simulink model "QcarModel_RoadExcitation_R2023a"  (R2023b)
settings: Solver=FixedStepAuto  StartTime=0.0  StopTime=5  FixedStep=0.01  RelTol=1e-3
values from neighbouring files (symbols this model uses):
  c = 20000    [QCarModel_Frequency_V2.m]    (also in QCarModel_Parameters.m)
  d = 1500    [QCarModel_Frequency_V2.m]    (also in QCarModel_Parameters.m)
  g = 981/100    (= 9.81)    [QCarModel_Frequency_V2.m]    (also in QCarModel_Parameters.m)
  m = mass(h)    [QCarModel_Frequency_V2.m]    (also in QCarModel_Parameters.m = 400)
settings Model: Creator=erona  LastModifiedBy=BeanieBabyJ
settings RTWCC: GPUComputeCapability=5.0

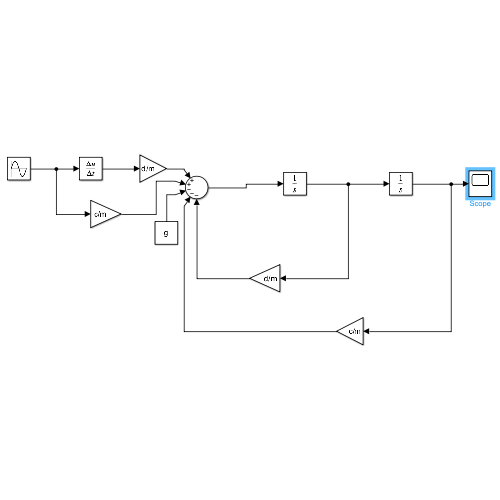
[thumbnail: Simulink's stored preview of the top-level diagram]
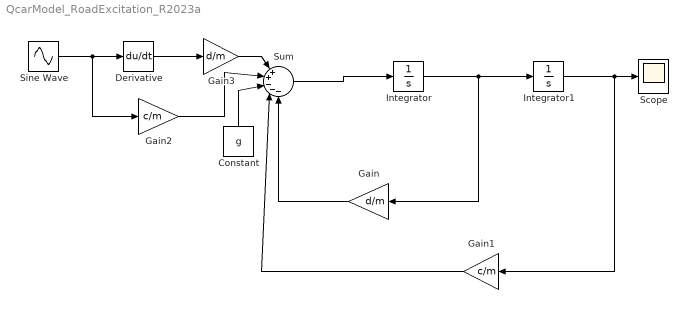
== system QcarModel_RoadExcitation_R2023a ==
  Constant : Constant  Value=g
  Derivative : Derivative
  Gain : Gain  Gain=d/m
  Gain1 : Gain  Gain=c/m
  Gain2 : Gain  Gain=c/m
  Gain3 : Gain  Gain=d/m
  Integrator : Integrator
  Integrator1 : Integrator
  Scope : Scope
  Sine Wave : Sin  Amplitude=0.02  Frequency=2*pi*100  Phase=pi/2  SampleTime=0
  Sum : Sum  Inputs=|++---
  wires:
  Integrator/1 -> Gain/1, Integrator1/1
  Sum/1 -> Integrator/1
  Integrator1/1 -> Scope/1, Gain1/1
  Constant/1 -> Sum/3
  Gain/1 -> Sum/5
  Gain1/1 -> Sum/4
  Derivative/1 -> Gain3/1
  Gain3/1 -> Sum/1
  Sine Wave/1 -> Derivative/1, Gain2/1
  Gain2/1 -> Sum/2
